simulink model "logical_oper"  (R2021a)
settings: Solver=VariableStepAuto  StartTime=0.0  StopTime=10.0  RelTol=1e-3
libraries: simulink x3
settings Model: Creator=lenovo  LastModifiedBy=lenovo

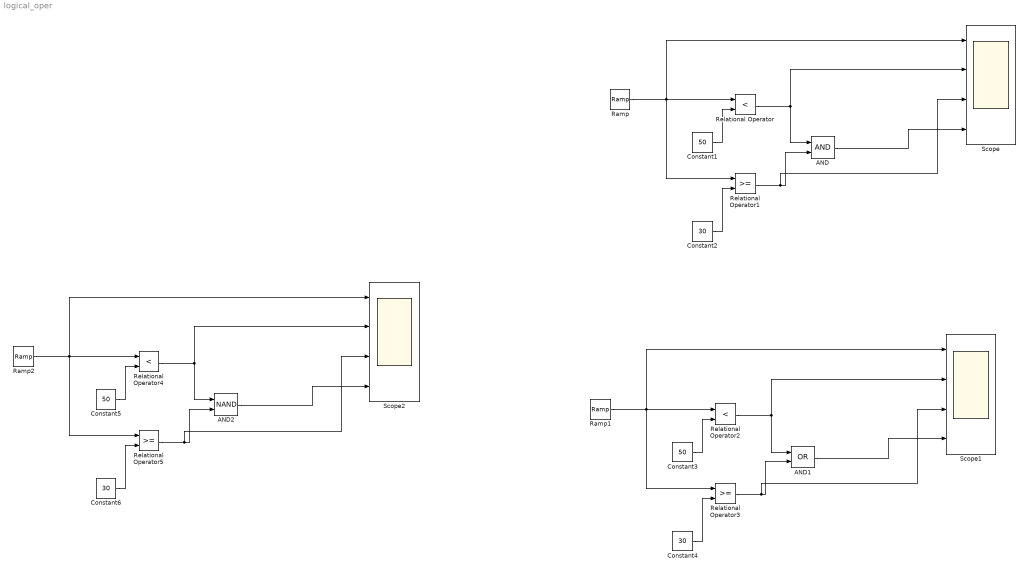
== system logical_oper ==
  AND : Logic  AllPortsSameDT=off  OutDataTypeStr=boolean
  AND1 : Logic  Operator=OR  AllPortsSameDT=off  OutDataTypeStr=boolean
  AND2 : Logic  Operator=NAND  AllPortsSameDT=off  OutDataTypeStr=boolean
  Constant1 : Constant  Value=50
  Constant2 : Constant  Value=30
  Constant3 : Constant  Value=50
  Constant4 : Constant  Value=30
  Constant5 : Constant  Value=50
  Constant6 : Constant  Value=30
  Ramp : simulink/Sources/Ramp  slope=1  start=0  InitialOutput=25
  Ramp1 : simulink/Sources/Ramp  slope=1  start=0  InitialOutput=25
  Ramp2 : simulink/Sources/Ramp  slope=1  start=0  InitialOutput=25
  Relational Operator : RelationalOperator  Operator=<  OutDataTypeStr=boolean  RndMeth=Simplest
  Relational Operator1 : RelationalOperator  OutDataTypeStr=boolean  RndMeth=Simplest
  Relational Operator2 : RelationalOperator  Operator=<  OutDataTypeStr=boolean  RndMeth=Simplest
  Relational Operator3 : RelationalOperator  OutDataTypeStr=boolean  RndMeth=Simplest
  Relational Operator4 : RelationalOperator  Operator=<  OutDataTypeStr=boolean  RndMeth=Simplest
  Relational Operator5 : RelationalOperator  OutDataTypeStr=boolean  RndMeth=Simplest
  Scope : Scope  NumInputPorts=4
  Scope1 : Scope  NumInputPorts=4
  Scope2 : Scope  NumInputPorts=4
  wires:
  Constant1/1 -> Relational Operator/2
  Constant2/1 -> Relational Operator1/2
  Ramp/1 -> Scope/1, Relational Operator1/1, Relational Operator/1
  Relational Operator/1 -> Scope/2, AND/1
  Relational Operator1/1 -> Scope/3, AND/2
  AND/1 -> Scope/4
  AND1/1 -> Scope1/4
  Relational Operator3/1 -> AND1/2, Scope1/3
  Relational Operator2/1 -> AND1/1, Scope1/2
  Ramp1/1 -> Relational Operator2/1, Relational Operator3/1, Scope1/1
  Constant4/1 -> Relational Operator3/2
  Constant3/1 -> Relational Operator2/2
  Constant5/1 -> Relational Operator4/2
  Constant6/1 -> Relational Operator5/2
  Ramp2/1 -> Scope2/1, Relational Operator5/1, Relational Operator4/1
  Relational Operator4/1 -> Scope2/2, AND2/1
  Relational Operator5/1 -> Scope2/3, AND2/2
  AND2/1 -> Scope2/4
